simulink model "valutazione_Kcr_Tcr"  (R2021b)
settings: Solver=VariableStepAuto  StartTime=0.0  StopTime=100  RelTol=1e-3
values from neighbouring files (symbols this model uses):
  r = 1    [script.m]
libraries: cstblocks x1
settings Model: Creator=antony  LastModifiedBy=antony

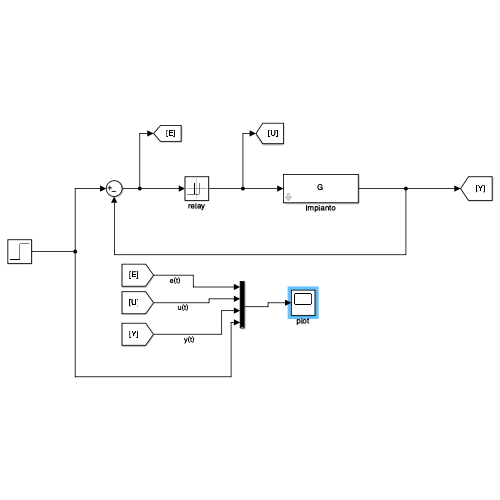
[thumbnail: Simulink's stored preview of the top-level diagram]
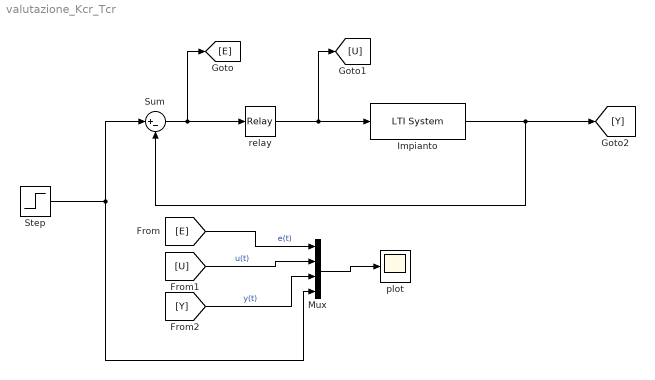
== system valutazione_Kcr_Tcr ==
  Impianto : cstblocks/LTI System  sys=G  IC=[]
  Mux : Mux
  Step : Step  Time=0  After=r  SampleTime=0
  Sum : Sum  Inputs=|+-
  plot : Scope
  relay : Relay  OnOutputValue=r  OffOutputValue=-r
  wires:
  Sum/1 -> [E], relay/1
  relay/1 -> [U], Impianto/1
  Impianto/1 -> [Y], Sum/2
  Mux/1 -> plot/1
  [E] -> Mux/1  "e(t)"
  [U] -> Mux/2  "u(t)"
  [Y] -> Mux/3  "y(t)"
  Step/1 -> Sum/1, Mux/4
